simulink model "calcul_vitesse_roues"  (R2024b)
settings: Solver=VariableStepAuto  StartTime=0.0  StopTime=10.0  RelTol=1e-3
values from neighbouring files (symbols this model uses):
  J = 0.5    [main_data_vehicle.m]
  Re = 0.47/2    (= 0.235)    [main_data_vehicle.m]
settings Model: Creator=marti  LastModifiedBy=marti

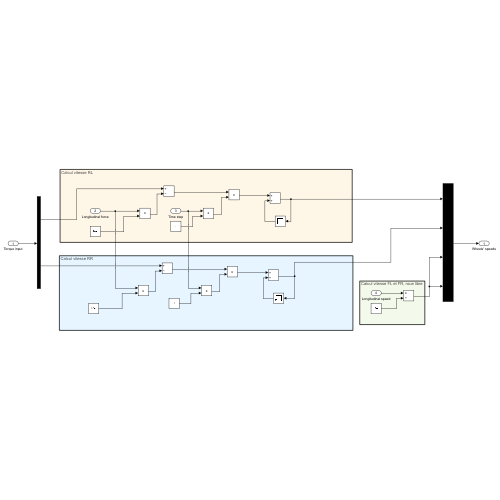
[thumbnail: Simulink's stored preview of the top-level diagram]
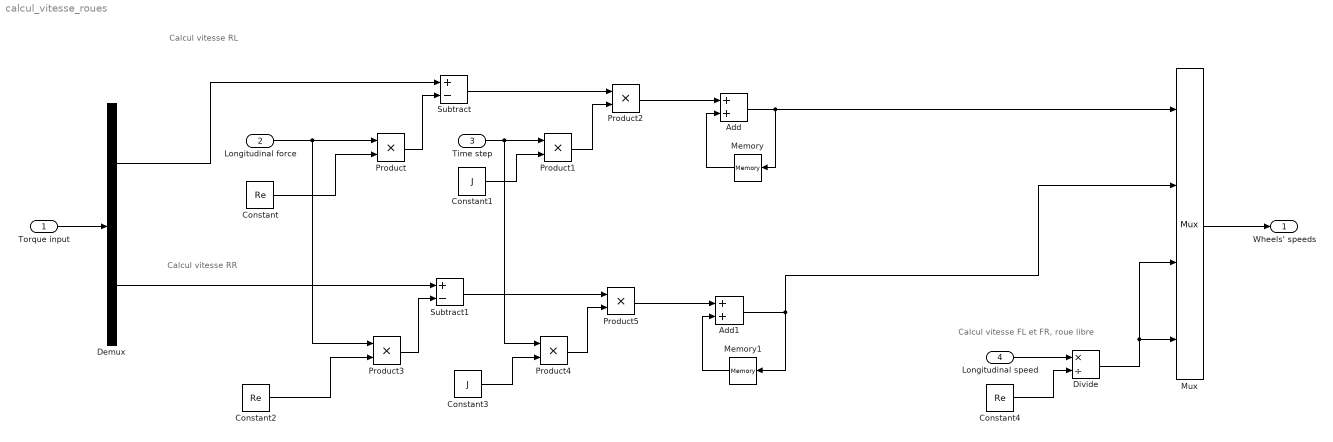
== system calcul_vitesse_roues ==
  note: Calcul vitesse FL et FR, roue libre
  note: Calcul vitesse RL
  note: Calcul vitesse RR
  Torque input : Inport
  Longitudinal force : Inport  Port=2
  Time step : Inport  Port=3
  Longitudinal speed : Inport  Port=4
  Add : Sum
  Add1 : Sum
  Constant : Constant  Value=Re
  Constant1 : Constant  Value=J
  Constant2 : Constant  Value=Re
  Constant3 : Constant  Value=J
  Constant4 : Constant  Value=Re
  Demux : Demux  Outputs=2
  Divide : Product  Inputs=*/
  Memory : Memory
  Memory1 : Memory
  Mux : Mux
  Product{,1..5} (6 alike) : Product
  Subtract : Sum  Inputs=+-
  Subtract1 : Sum  Inputs=+-
  Wheels' speeds : Outport
  wires:
  Constant/1 -> Product/2
  Longitudinal force/1 -> Product3/1, Product/1
  Product/1 -> Subtract/2
  Constant1/1 -> Product1/2
  Time step/1 -> Product4/1, Product1/1
  Product1/1 -> Product2/2
  Subtract/1 -> Product2/1
  Product2/1 -> Add/1
  Add/1 -> Mux/1, Memory/1
  Memory/1 -> Add/2
  Torque input/1 -> Demux/1
  Subtract1/1 -> Product5/1
  Constant3/1 -> Product4/2
  Constant2/1 -> Product3/2
  Product4/1 -> Product5/2
  Add1/1 -> Mux/2, Memory1/1
  Memory1/1 -> Add1/2
  Product3/1 -> Subtract1/2
  Product5/1 -> Add1/1
  Demux/2 -> Subtract1/1
  Demux/1 -> Subtract/1
  Longitudinal speed/1 -> Divide/1
  Constant4/1 -> Divide/2
  Divide/1 -> Mux/4, Mux/3
  Mux/1 -> Wheels' speeds/1
